simulink model "HP_Filter"  (Simulink 7.4)
settings: Solver=ode45  StartTime=0.0  StopTime=10.0  RelTol=1e-3
values from neighbouring files (symbols this model uses):
  Ts = 0.005    [quadrocopter_param.m]
undefined symbols (not defined in the file or in its folder): DiscIntNeverNeededParam, K
settings Model: Creator=roczit00  LastModifiedBy=roczit00

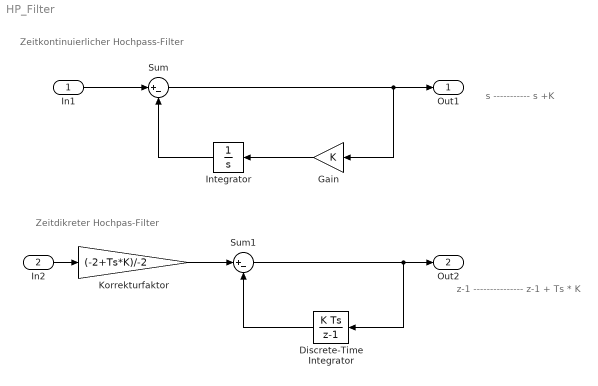
== system HP_Filter ==
  note: Zeitkontinuierlicher Hochpass-Filter
  note: s
      | -----------
      | s +K
  note: Zeitdikreter Hochpas-Filter
  note: z-1
      | ---------------
      | z-1 + Ts * K
  In1 : Inport  OutDataType=fixdt(1, 16)  OutScaling=2^0
  In2 : Inport  Port=2  OutDataType=fixdt(1, 16)  OutScaling=2^0
  Discrete-Time Integrator : DiscreteIntegrator  OutDataType=fixdt(1, 16)  OutScaling=2^0  ICPrevOutput=DiscIntNeverNeededParam  ICPrevScaledInput=DiscIntNeverNeededParam
  Gain : Gain  Gain=K  ParameterDataType=fixdt(1, 16)  ParameterScaling=2^0  OutDataType=fixdt(1, 16)  OutScaling=2^0
  Integrator : Integrator
  Korrekturfaktor : Gain  Gain=(-2+Ts*K)/-2  ParameterDataType=fixdt(1, 16)  ParameterScaling=2^0  OutDataType=fixdt(1, 16)  OutScaling=2^0
  Sum : Sum  Inputs=|+-  OutDataType=fixdt(1, 16)  OutScaling=2^0
  Sum1 : Sum  Inputs=|+-  OutDataType=fixdt(1, 16)  OutScaling=2^0
  Out1 : Outport  OutDataType=fixdt(1, 16)  OutScaling=2^0
  Out2 : Outport  Port=2  OutDataType=fixdt(1, 16)  OutScaling=2^0
  wires:
  In1/1 -> Sum/1
  Integrator/1 -> Sum/2
  Sum/1 -> Out1/1, Gain/1
  Gain/1 -> Integrator/1
  Discrete-Time Integrator/1 -> Sum1/2
  Sum1/1 -> Out2/1, Discrete-Time Integrator/1
  In2/1 -> Korrekturfaktor/1
  Korrekturfaktor/1 -> Sum1/1
